simulink model "Battery_Model"  (R2016b)
settings: Solver=ode1  StartTime=0.0  StopTime=1180  FixedStep=0.1  RelTol=1e-3
InitFcn:
  | init_soc=0.6;
values from neighbouring files (symbols this model uses):
  C1_charge = C1_discharge    [Batt_init.m]
  C1_discharge = [54.148429	21.802633	25.586141	30.914925	26.854337	32.525752	40.18035	1.503165	44.76751	43.347833	43.347833 ... (first row only)    [Batt_init.m]
  R0_charge = R0_discharge    [Batt_init.m]
  R0_discharge = [0.0771	0.0168	0.0135	0.0123	0.0117	0.0123	0.0117	0.012	0.0117	0.0114	0.012 ... (first row only)    [Batt_init.m]
  R1_charge = [0.032155	0.008199	0.004763	0.004183	0.00348	0.003242	0.003193	0.003006	0.003091	0.003062	0.003062 ... (first row only)    [Batt_init.m]
  SOC = [0 0.1 0.2 0.3 0.4 0.5 0.6 0.7 0.8 0.9 1]    [Batt_init.m]
  Voc_charge = [2.59 3.22 3.26 3.3 3.3 3.31 3.31 3.32 3.34 3.34 3.47 ... (first row only)    [Batt_init.m]
  Voc_discharge = [2.66	3.19	3.23	3.26	3.28	3.28	3.29	3.3	3.33	3.33	3.4 ... (first row only)    [Batt_init.m]
undefined symbols (not defined in the file or in its folder): cell_capacity, Cp, Hysterisis, Mass_Batt, parallel_cells, series_cells
settings Model: Creator=vguturi  LastModifiedBy=vguturi

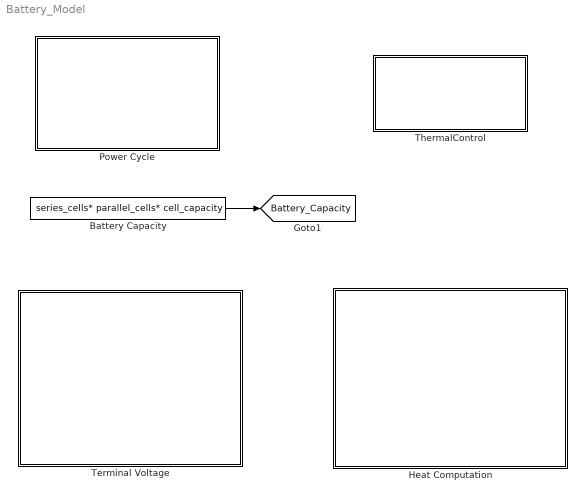
== system Battery_Model ==
  Battery Capacity : Constant  Value=series_cells* parallel_cells* cell_capacity
  Heat Computation : Subsystem  Variant=on  VariantControl=Variant1
  Power Cycle : Subsystem
  Terminal Voltage : Subsystem  Variant=on
  ThermalControl : Subsystem
  tag scope: Battery_Capacity=global
  wires:
  Battery Capacity/1 -> [Battery_Capacity]

== system Battery_Model/Heat Computation ==
  Heat Estimation SimpleR : Subsystem  VariantControl=HeatEst_SimpleR
  Heat Estimation TheveninRC : Subsystem  VariantControl=HeatEst_TheveninRC

== system Battery_Model/Power Cycle ==
  From Workspace : FromWorkspace  VariableName=NEDC
  Scope : Scope
  tag scope: Pd=global
  wires:
  From Workspace/1 -> Scope/1, [Pd]

== system Battery_Model/Terminal Voltage ==
  note: 1) Add Subsystem or Model blocks as valid variant choices.
      | 2) You cannot connect blocks at this level. At simulation, connectivity is automatically
      | determined, based on the active variant and port name matching.
  SimpleResistiveCircuit : Subsystem  VariantControl=SimpleResistive
  TheveninFirstOrder : Subsystem  VariantControl=TheveninRC

== system Battery_Model/ThermalControl ==
  Batt Temp Control : Stateflow chart  TreatAsAtomicUnit=on
  Hysterisis : Constant  Value=Hysterisis
  Scope : Scope  NumInputPorts=2
  tag scope: Cool_Cmd=global
  wires:
  Hysterisis/1 -> Batt Temp Control/1(hysterisis)
  [BattTemp] -> Scope/2, Batt Temp Control/2(Batt_Temp)
  Batt Temp Control/1(Cool_Cmd) -> Scope/1, [Cool_Cmd]

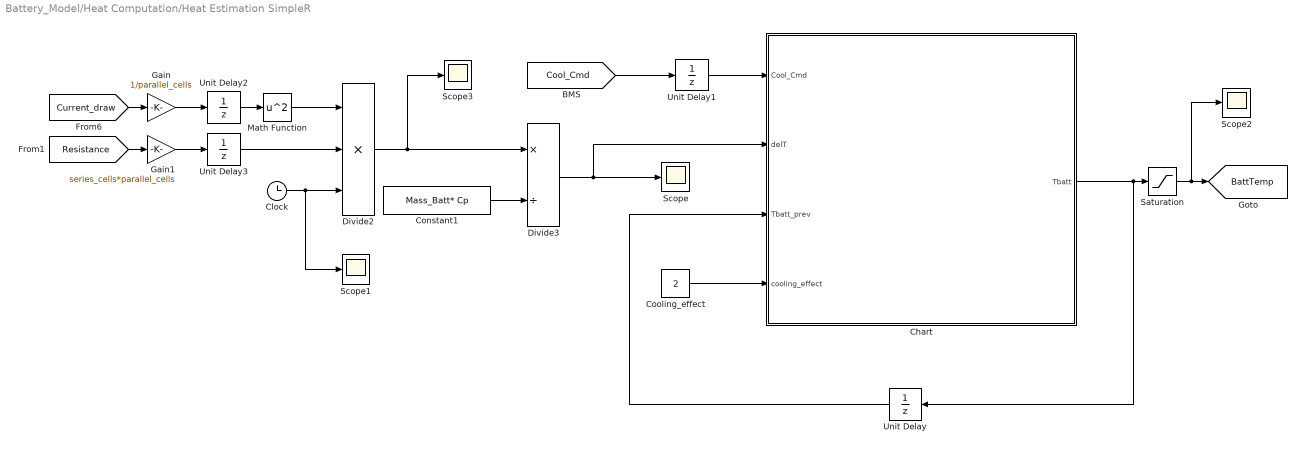
== system Battery_Model/Heat Computation/Heat Estimation SimpleR ==
  Chart : Stateflow chart  TreatAsAtomicUnit=on
  Clock : Clock
  Constant1 : Constant  Value=Mass_Batt* Cp
  Cooling_effect : Constant  Value=2
  Divide2 : Product  Inputs=***
  Divide3 : Product  Inputs=*/
  Gain : Gain  Gain=1/parallel_cells
  Gain1 : Gain  Gain=series_cells*parallel_cells
  Math Function : Math  Operator=square  SaturateOnIntegerOverflow=on
  Saturation : Saturate  UpperLimit=400  LowerLimit=250
  Scope{,1..3} (4 alike) : Scope
  Unit Delay : UnitDelay  InitialCondition=300  SampleTime=-1
  Unit Delay1 : UnitDelay  SampleTime=-1
  Unit Delay2 : UnitDelay  InitialCondition=10  SampleTime=-1
  Unit Delay3 : UnitDelay  InitialCondition=0.012  SampleTime=-1
  tag scope: BattTemp=global
  wires:
  Math Function/1 -> Divide2/1
  Divide2/1 -> Scope3/1, Divide3/1
  [Current_draw] -> Gain/1
  Clock/1 -> Scope1/1, Divide2/3
  Divide3/1 -> Scope/1, Chart/2(delT)
  Constant1/1 -> Divide3/2
  [Resistance] -> Gain1/1
  [Cool_Cmd] -> Unit Delay1/1
  Unit Delay/1 -> Chart/3(Tbatt_prev)
  Chart/1(Tbatt) -> Unit Delay/1, Saturation/1
  Unit Delay1/1 -> Chart/1(Cool_Cmd)
  Cooling_effect/1 -> Chart/4(cooling_effect)
  Unit Delay2/1 -> Math Function/1
  Unit Delay3/1 -> Divide2/2
  Gain/1 -> Unit Delay2/1
  Gain1/1 -> Unit Delay3/1
  Saturation/1 -> Scope2/1, [BattTemp]

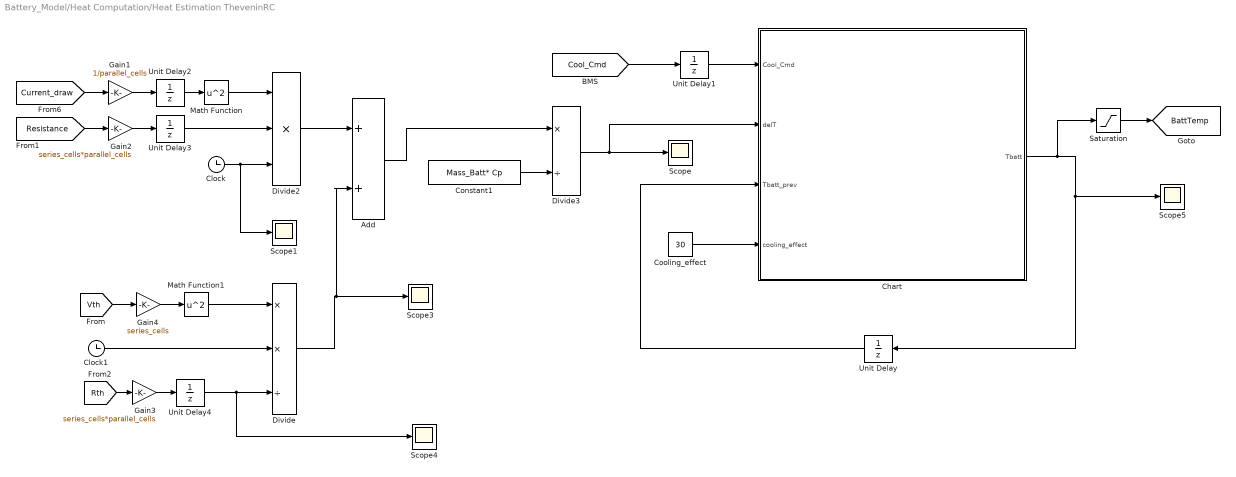
== system Battery_Model/Heat Computation/Heat Estimation TheveninRC ==
  Add : Sum
  Chart : Stateflow chart  TreatAsAtomicUnit=on
  Clock : Clock
  Clock1 : Clock
  Constant1 : Constant  Value=Mass_Batt* Cp
  Cooling_effect : Constant  Value=30
  Divide : Product  Inputs=**/
  Divide2 : Product  Inputs=***
  Divide3 : Product  Inputs=*/
  Gain1 : Gain  Gain=1/parallel_cells
  Gain2 : Gain  Gain=series_cells*parallel_cells
  Gain3 : Gain  Gain=series_cells*parallel_cells
  Gain4 : Gain  Gain=series_cells
  Math Function : Math  Operator=square  SaturateOnIntegerOverflow=on
  Math Function1 : Math  Operator=square  SaturateOnIntegerOverflow=on
  Saturation : Saturate  UpperLimit=400  LowerLimit=250
  Scope{,1,3..5} (5 alike) : Scope
  Unit Delay : UnitDelay  InitialCondition=300  SampleTime=-1
  Unit Delay1 : UnitDelay  SampleTime=-1
  Unit Delay2 : UnitDelay  SampleTime=-1
  Unit Delay3 : UnitDelay  InitialCondition=0.012  SampleTime=-1
  Unit Delay4 : UnitDelay  InitialCondition=0.012  SampleTime=-1
  tag scope: BattTemp=global
  wires:
  Math Function/1 -> Divide2/1
  [Current_draw] -> Gain1/1
  Clock/1 -> Scope1/1, Divide2/3
  Divide3/1 -> Scope/1, Chart/2(delT)
  Constant1/1 -> Divide3/2
  [Resistance] -> Gain2/1
  [Cool_Cmd] -> Unit Delay1/1
  Unit Delay/1 -> Chart/3(Tbatt_prev)
  Chart/1(Tbatt) -> Saturation/1, Scope5/1, Unit Delay/1
  Unit Delay1/1 -> Chart/1(Cool_Cmd)
  Cooling_effect/1 -> Chart/4(cooling_effect)
  Unit Delay2/1 -> Math Function/1
  Unit Delay3/1 -> Divide2/2
  [Vth] -> Gain4/1
  Math Function1/1 -> Divide/1
  [Rth] -> Gain3/1
  Clock1/1 -> Divide/2
  Unit Delay4/1 -> Scope4/1, Divide/3
  Divide2/1 -> Add/1
  Add/1 -> Divide3/1
  Divide/1 -> Add/2, Scope3/1
  Gain2/1 -> Unit Delay3/1
  Gain1/1 -> Unit Delay2/1
  Gain3/1 -> Unit Delay4/1
  Gain4/1 -> Math Function1/1
  Saturation/1 -> [BattTemp]

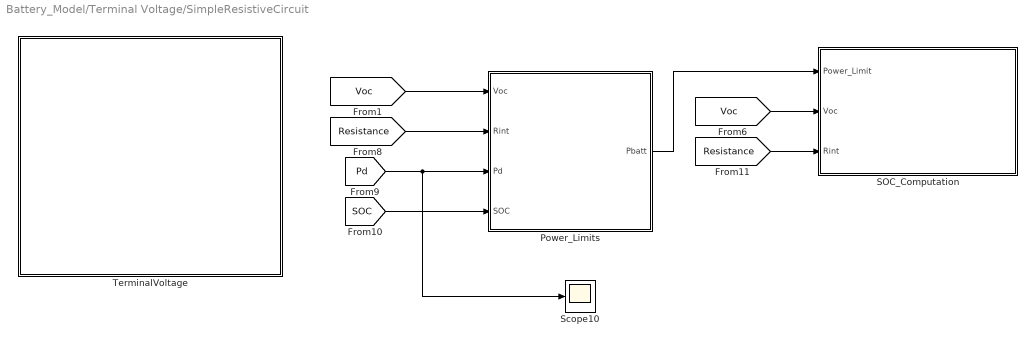
== system Battery_Model/Terminal Voltage/SimpleResistiveCircuit ==
  Power_Limits : Subsystem
  SOC_Computation : Subsystem
  Scope10 : Scope
  TerminalVoltage : Subsystem
  wires:
  [Resistance] -> Power_Limits/2(Rint)
  [Pd] -> Scope10/1, Power_Limits/3(Pd)
  [SOC] -> Power_Limits/4(SOC)
  [Resistance] -> SOC_Computation/3(Rint)
  [Voc] -> Power_Limits/1(Voc)
  [Voc] -> SOC_Computation/2(Voc)
  Power_Limits/1(Pbatt) -> SOC_Computation/1(Power_Limit)

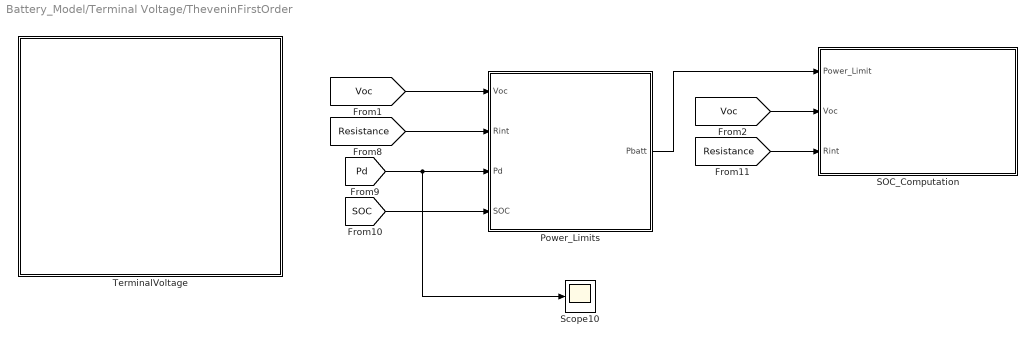
== system Battery_Model/Terminal Voltage/TheveninFirstOrder ==
  Power_Limits : Subsystem
  SOC_Computation : Subsystem
  Scope10 : Scope
  TerminalVoltage : Subsystem
  wires:
  [Resistance] -> Power_Limits/2(Rint)
  [Pd] -> Scope10/1, Power_Limits/3(Pd)
  [SOC] -> Power_Limits/4(SOC)
  [Resistance] -> SOC_Computation/3(Rint)
  [Voc] -> Power_Limits/1(Voc)
  [Voc] -> SOC_Computation/2(Voc)
  Power_Limits/1(Pbatt) -> SOC_Computation/1(Power_Limit)

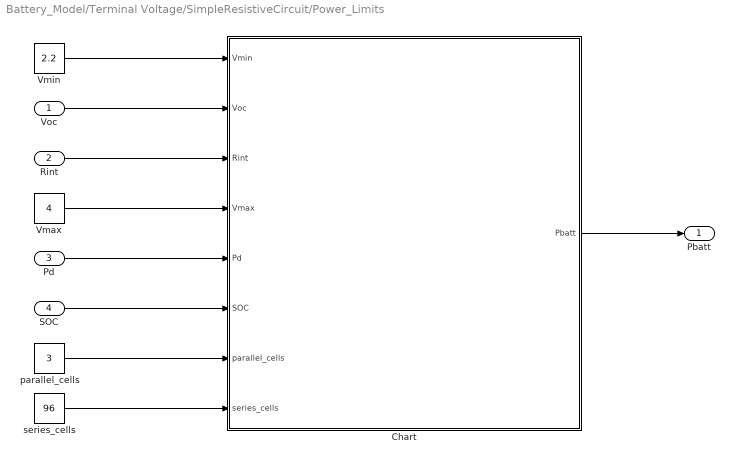
== system Battery_Model/Terminal Voltage/SimpleResistiveCircuit/Power_Limits ==
  Voc : Inport
  Rint : Inport  Port=2
  Pd : Inport  Port=3
  SOC : Inport  Port=4
  Chart : Stateflow chart  TreatAsAtomicUnit=on
  Vmax : Constant  Value=4
  Vmin : Constant  Value=2.2
  parallel_cells : Constant  Value=3
  series_cells : Constant  Value=96
  Pbatt : Outport
  wires:
  Vmin/1 -> Chart/1(Vmin)
  Vmax/1 -> Chart/4(Vmax)
  Voc/1 -> Chart/2(Voc)
  Rint/1 -> Chart/3(Rint)
  Pd/1 -> Chart/5(Pd)
  SOC/1 -> Chart/6(SOC)
  Chart/1(Pbatt) -> Pbatt/1
  series_cells/1 -> Chart/8(series_cells)
  parallel_cells/1 -> Chart/7(parallel_cells)

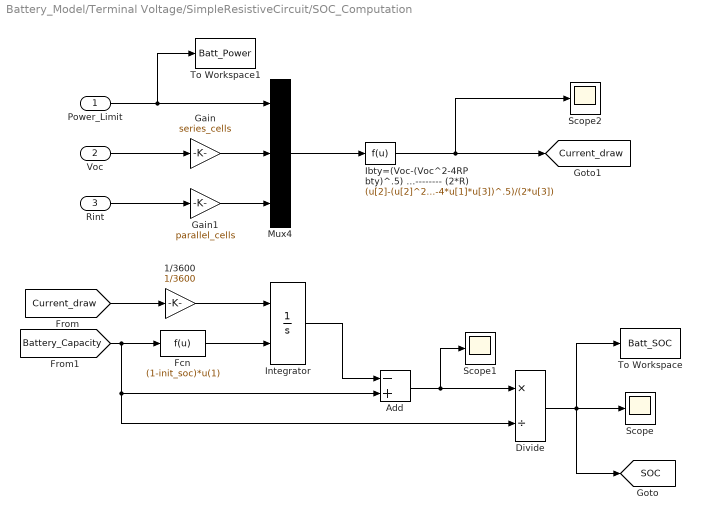
== system Battery_Model/Terminal Voltage/SimpleResistiveCircuit/SOC_Computation ==
  Power_Limit : Inport
  Voc : Inport  Port=2
  Rint : Inport  Port=3
  1/3600 : Gain  Gain=1/3600
  Add : Sum  Inputs=-+
  Divide : Product  Inputs=*/
  Fcn : Fcn  Expr=(1-init_soc)*u(1)
  Gain : Gain  Gain=series_cells
  Gain1 : Gain  Gain=parallel_cells
  Ibty=(Voc-(Voc^2-4RPbty)^.5) ----------------------------- (2*R) : Fcn  Expr=(u[2]-(u[2]^2-4*u[1]*u[3])^.5)/(2*u[3])
  Integrator : Integrator  InitialConditionSource=external
  Mux4 : Mux  Inputs=3
  Scope : Scope
  Scope1 : Scope
  Scope2 : Scope
  To Workspace : ToWorkspace  VariableName=Batt_SOC  SaveFormat=Timeseries  SampleTime=-1
  To Workspace1 : ToWorkspace  VariableName=Batt_Power  SaveFormat=Timeseries  SampleTime=-1
  tag scope: Current_draw=global, SOC=global
  wires:
  1/3600/1 -> Integrator/1
  [Current_draw] -> 1/3600/1
  [Battery_Capacity] -> Fcn/1, Divide/2, Add/2
  Add/1 -> Scope1/1, Divide/1
  Divide/1 -> To Workspace/1, [SOC], Scope/1
  Integrator/1 -> Add/1
  Fcn/1 -> Integrator/2
  Mux4/1 -> Ibty=(Voc-(Voc^2-4RPbty)^.5) ----------------------------- (2*R)/1
  Gain/1 -> Mux4/2
  Gain1/1 -> Mux4/3
  Ibty=(Voc-(Voc^2-4RPbty)^.5) ----------------------------- (2*R)/1 -> Scope2/1, [Current_draw]
  Power_Limit/1 -> To Workspace1/1, Mux4/1
  Voc/1 -> Gain/1
  Rint/1 -> Gain1/1

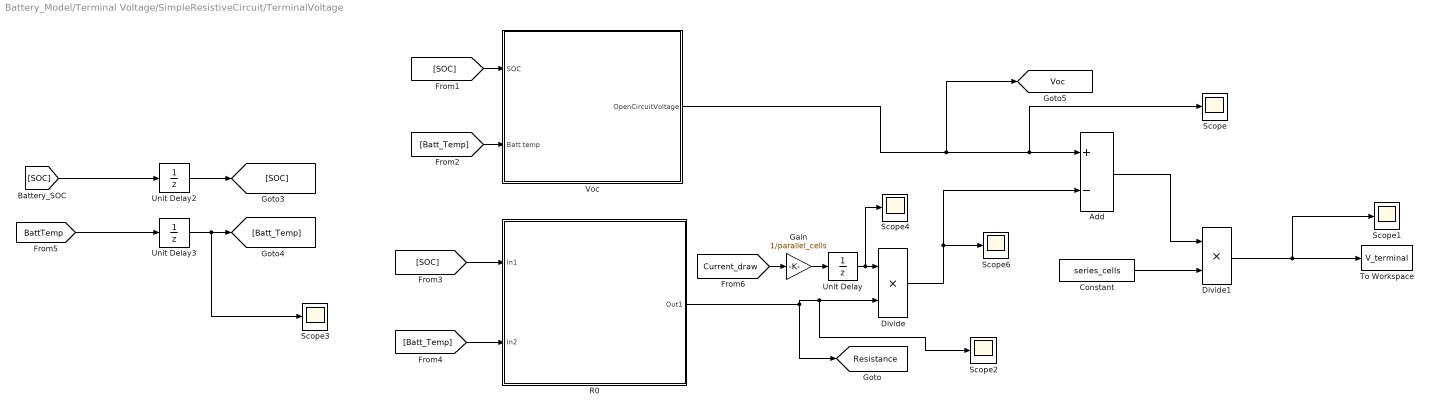
== system Battery_Model/Terminal Voltage/SimpleResistiveCircuit/TerminalVoltage ==
  Add : Sum  Inputs=+-
  Constant : Constant  Value=series_cells
  Divide : Product  Inputs=**
  Divide1 : Product  Inputs=**
  Gain : Gain  Gain=1/parallel_cells
  R0 : Subsystem
  Scope{,1..4,6} (6 alike) : Scope
  To Workspace : ToWorkspace  VariableName=V_terminal  SaveFormat=Timeseries  SampleTime=-1
  Unit Delay : UnitDelay  SampleTime=-1
  Unit Delay2 : UnitDelay  InitialCondition=0.6  SampleTime=-1
  Unit Delay3 : UnitDelay  InitialCondition=300  SampleTime=-1
  Voc : Subsystem
  tag scope: Resistance=global, Voc=global
  wires:
  [SOC] -> Voc/1(SOC)
  [Batt_Temp] -> Voc/2(Batt temp)
  Unit Delay/1 -> Scope4/1, Divide/1
  Add/1 -> Divide1/1
  Divide1/1 -> Scope1/1, To Workspace/1
  Divide/1 -> Scope6/1, Add/2
  Constant/1 -> Divide1/2
  R0/1(Out1) -> Scope2/1, Divide/2, [Resistance]
  [BattTemp] -> Unit Delay3/1
  [SOC] -> Unit Delay2/1
  Unit Delay2/1 -> [SOC]
  Unit Delay3/1 -> Scope3/1, [Batt_Temp]
  [SOC] -> R0/1(In1)
  [Batt_Temp] -> R0/2(In2)
  Voc/1(OpenCircuitVoltage) -> [Voc], Scope/1, Add/1
  [Current_draw] -> Gain/1
  Gain/1 -> Unit Delay/1

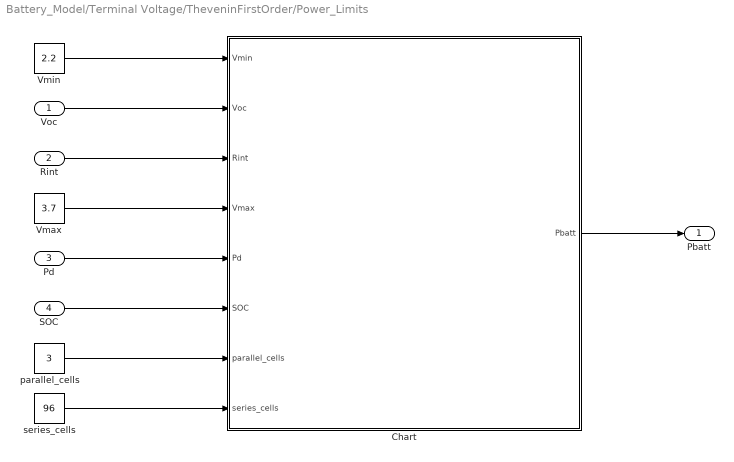
== system Battery_Model/Terminal Voltage/TheveninFirstOrder/Power_Limits ==
  Voc : Inport
  Rint : Inport  Port=2
  Pd : Inport  Port=3
  SOC : Inport  Port=4
  Chart : Stateflow chart  TreatAsAtomicUnit=on
  Vmax : Constant  Value=3.7
  Vmin : Constant  Value=2.2
  parallel_cells : Constant  Value=3
  series_cells : Constant  Value=96
  Pbatt : Outport
  wires:
  Vmin/1 -> Chart/1(Vmin)
  Vmax/1 -> Chart/4(Vmax)
  Voc/1 -> Chart/2(Voc)
  Rint/1 -> Chart/3(Rint)
  Pd/1 -> Chart/5(Pd)
  SOC/1 -> Chart/6(SOC)
  Chart/1(Pbatt) -> Pbatt/1
  series_cells/1 -> Chart/8(series_cells)
  parallel_cells/1 -> Chart/7(parallel_cells)

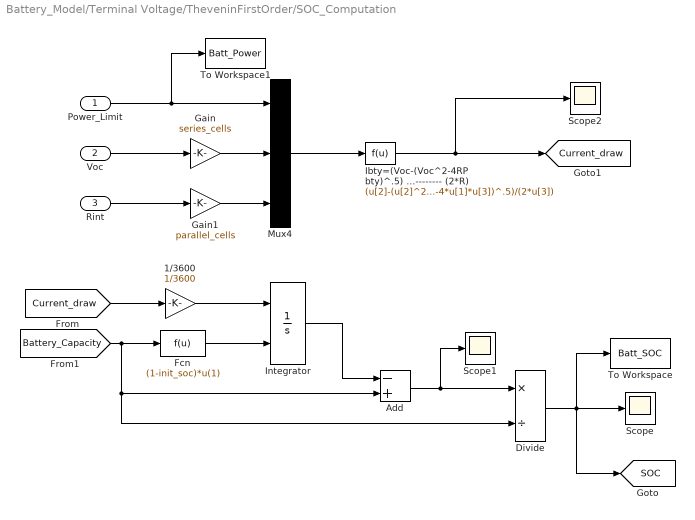
== system Battery_Model/Terminal Voltage/TheveninFirstOrder/SOC_Computation ==
  Power_Limit : Inport
  Voc : Inport  Port=2
  Rint : Inport  Port=3
  1/3600 : Gain  Gain=1/3600
  Add : Sum  Inputs=-+
  Divide : Product  Inputs=*/
  Fcn : Fcn  Expr=(1-init_soc)*u(1)
  Gain : Gain  Gain=series_cells
  Gain1 : Gain  Gain=parallel_cells
  Ibty=(Voc-(Voc^2-4RPbty)^.5) ----------------------------- (2*R) : Fcn  Expr=(u[2]-(u[2]^2-4*u[1]*u[3])^.5)/(2*u[3])
  Integrator : Integrator  InitialConditionSource=external
  Mux4 : Mux  Inputs=3
  Scope : Scope
  Scope1 : Scope
  Scope2 : Scope
  To Workspace : ToWorkspace  VariableName=Batt_SOC  SaveFormat=Timeseries  SampleTime=-1
  To Workspace1 : ToWorkspace  VariableName=Batt_Power  SaveFormat=Timeseries  SampleTime=-1
  tag scope: Current_draw=global, SOC=global
  wires:
  1/3600/1 -> Integrator/1
  [Current_draw] -> 1/3600/1
  [Battery_Capacity] -> Fcn/1, Divide/2, Add/2
  Add/1 -> Scope1/1, Divide/1
  Divide/1 -> To Workspace/1, [SOC], Scope/1
  Integrator/1 -> Add/1
  Fcn/1 -> Integrator/2
  Mux4/1 -> Ibty=(Voc-(Voc^2-4RPbty)^.5) ----------------------------- (2*R)/1
  Gain/1 -> Mux4/2
  Gain1/1 -> Mux4/3
  Ibty=(Voc-(Voc^2-4RPbty)^.5) ----------------------------- (2*R)/1 -> Scope2/1, [Current_draw]
  Power_Limit/1 -> To Workspace1/1, Mux4/1
  Voc/1 -> Gain/1
  Rint/1 -> Gain1/1

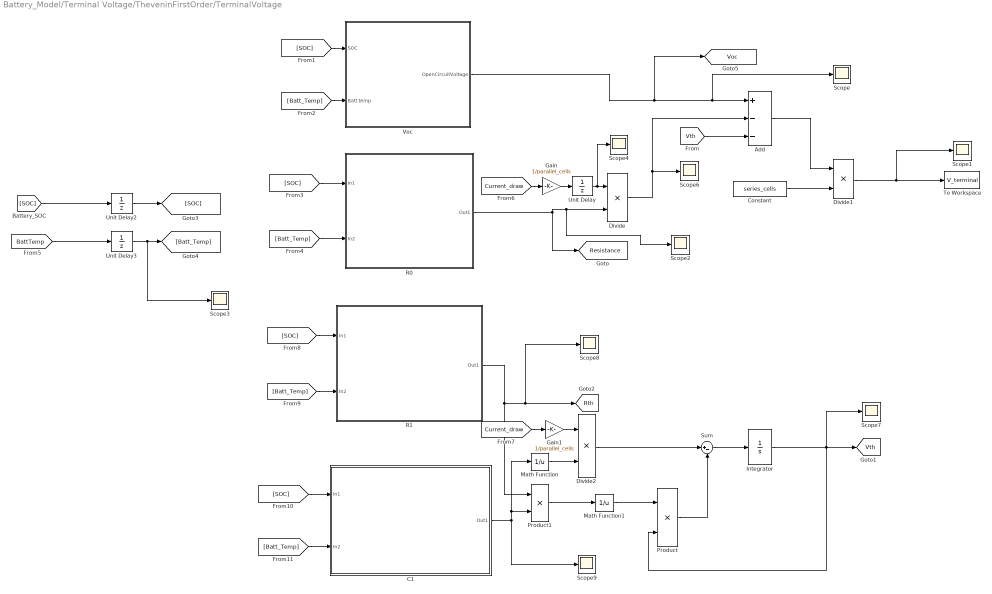
== system Battery_Model/Terminal Voltage/TheveninFirstOrder/TerminalVoltage ==
  Add : Sum  Inputs=+--
  C1 : Subsystem
  Constant : Constant  Value=series_cells
  Divide : Product  Inputs=**
  Divide1 : Product  Inputs=**
  Divide2 : Product  Inputs=**
  Gain : Gain  Gain=1/parallel_cells
  Gain1 : Gain  Gain=1/parallel_cells
  Integrator : Integrator
  Math Function : Math  Operator=reciprocal  SaturateOnIntegerOverflow=on
  Math Function1 : Math  Operator=reciprocal  SaturateOnIntegerOverflow=on
  Product : Product
  Product1 : Product
  R0 : Subsystem
  R1 : Subsystem
  Scope{,1..4,6..9} (9 alike) : Scope
  Sum : Sum  Inputs=|+-
  To Workspace : ToWorkspace  VariableName=V_terminal  SaveFormat=Timeseries  SampleTime=-1
  Unit Delay : UnitDelay  SampleTime=-1
  Unit Delay2 : UnitDelay  InitialCondition=0.6  SampleTime=-1
  Unit Delay3 : UnitDelay  InitialCondition=300  SampleTime=-1
  Voc : Subsystem
  tag scope: Resistance=global, Rth=global, Voc=global, Vth=global
  wires:
  [SOC] -> R1/1(In1)
  [SOC] -> Voc/1(SOC)
  [Batt_Temp] -> Voc/2(Batt temp)
  [Batt_Temp] -> R1/2(In2)
  Unit Delay/1 -> Scope4/1, Divide/1
  Add/1 -> Divide1/1
  Divide1/1 -> Scope1/1, To Workspace/1
  Divide/1 -> Scope6/1, Add/2
  Constant/1 -> Divide1/2
  Integrator/1 -> Scope7/1, [Vth], Product/2
  [Current_draw] -> Gain1/1
  Math Function/1 -> Divide2/2
  [Vth] -> Add/3
  Product1/1 -> Math Function1/1
  Product/1 -> Sum/2
  Math Function1/1 -> Product/1
  Sum/1 -> Integrator/1
  Divide2/1 -> Sum/1
  R0/1(Out1) -> Scope2/1, Divide/2, [Resistance]
  R1/1(Out1) -> Product1/1, Scope8/1, [Rth]
  C1/1(Out1) -> Scope9/1, Math Function/1, Product1/2
  [BattTemp] -> Unit Delay3/1
  [SOC] -> Unit Delay2/1
  Unit Delay2/1 -> [SOC]
  Unit Delay3/1 -> Scope3/1, [Batt_Temp]
  [SOC] -> R0/1(In1)
  [Batt_Temp] -> R0/2(In2)
  [SOC] -> C1/1(In1)
  [Batt_Temp] -> C1/2(In2)
  Voc/1(OpenCircuitVoltage) -> [Voc], Scope/1, Add/1
  [Current_draw] -> Gain/1
  Gain/1 -> Unit Delay/1
  Gain1/1 -> Divide2/1

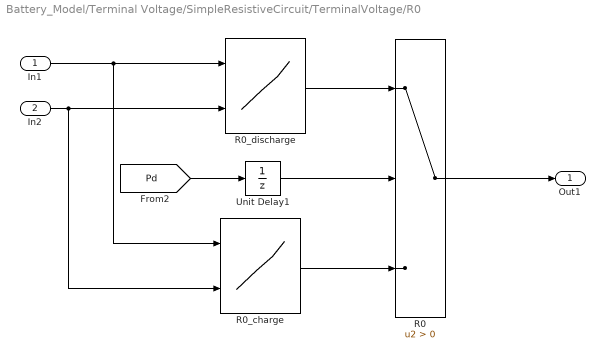
== system Battery_Model/Terminal Voltage/SimpleResistiveCircuit/TerminalVoltage/R0 ==
  In1 : Inport
  In2 : Inport  Port=2
  R0 : Switch  Criteria=u2 > Threshold
  R0_charge : Lookup_n-D  BreakpointsForDimension1=[293 303 313]  BreakpointsForDimension2=SOC  Table=R0_charge  ExtrapMethod=Clip  UseLastTableValue=on  InternalRulePriority=Speed  RndMeth=Simplest  InputSameDT=on
  R0_discharge : Lookup_n-D  BreakpointsForDimension1=[293 303 313]  BreakpointsForDimension2=SOC  Table=R0_discharge  ExtrapMethod=Clip  UseLastTableValue=on  InternalRulePriority=Speed  RndMeth=Simplest  InputSameDT=on
  Unit Delay1 : UnitDelay  SampleTime=-1
  Out1 : Outport
  wires:
  [Pd] -> Unit Delay1/1
  Unit Delay1/1 -> R0/2
  R0_discharge/1 -> R0/1
  R0_charge/1 -> R0/3
  R0/1 -> Out1/1
  In1/1 -> R0_charge/1, R0_discharge/1
  In2/1 -> R0_charge/2, R0_discharge/2

== system Battery_Model/Terminal Voltage/SimpleResistiveCircuit/TerminalVoltage/Voc ==
  SOC : Inport
  Batt temp : Inport  Port=2
  Voc : Switch  Criteria=u2 > Threshold
  Voc_charge : Lookup_n-D  BreakpointsForDimension1=[293 303 313]  BreakpointsForDimension2=SOC  Table=Voc_charge  ExtrapMethod=Clip  UseLastTableValue=on  InternalRulePriority=Speed  RndMeth=Simplest  InputSameDT=on
  Voc_discharge : Lookup_n-D  BreakpointsForDimension1=[293 303 313]  BreakpointsForDimension2=SOC  Table=Voc_discharge  ExtrapMethod=Clip  UseLastTableValue=on  InternalRulePriority=Speed  RndMeth=Simplest  InputSameDT=on
  OpenCircuitVoltage : Outport
  wires:
  Batt temp/1 -> Voc_charge/2, Voc_discharge/2
  SOC/1 -> Voc_discharge/1, Voc_charge/1
  Voc_charge/1 -> Voc/3
  Voc/1 -> OpenCircuitVoltage/1
  [Pd] -> Voc/2
  Voc_discharge/1 -> Voc/1

== system Battery_Model/Terminal Voltage/TheveninFirstOrder/TerminalVoltage/C1 ==
  In1 : Inport
  In2 : Inport  Port=2
  C1 : Switch  Criteria=u2 > Threshold
  C1_charge : Lookup_n-D  BreakpointsForDimension1=[293 303 313]  BreakpointsForDimension2=SOC  Table=C1_charge  ExtrapMethod=Clip  UseLastTableValue=on  InternalRulePriority=Speed  RndMeth=Simplest  InputSameDT=on
  C1_discharge : Lookup_n-D  BreakpointsForDimension1=[293 303 313]  BreakpointsForDimension2=SOC  Table=C1_discharge  ExtrapMethod=Clip  UseLastTableValue=on  InternalRulePriority=Speed  RndMeth=Simplest  InputSameDT=on
  Unit Delay5 : UnitDelay  SampleTime=-1
  Out1 : Outport
  wires:
  [Pd] -> Unit Delay5/1
  Unit Delay5/1 -> C1/2
  C1_discharge/1 -> C1/1
  C1_charge/1 -> C1/3
  C1/1 -> Out1/1
  In1/1 -> C1_charge/1, C1_discharge/1
  In2/1 -> C1_charge/2, C1_discharge/2

== system Battery_Model/Terminal Voltage/TheveninFirstOrder/TerminalVoltage/R0 ==
  In1 : Inport
  In2 : Inport  Port=2
  R0 : Switch  Criteria=u2 > Threshold
  R0_charge : Lookup_n-D  BreakpointsForDimension1=[293 303 313]  BreakpointsForDimension2=SOC  Table=R0_charge  ExtrapMethod=Clip  UseLastTableValue=on  InternalRulePriority=Speed  RndMeth=Simplest  InputSameDT=on
  R0_discharge : Lookup_n-D  BreakpointsForDimension1=[293 303 313]  BreakpointsForDimension2=SOC  Table=R0_discharge  ExtrapMethod=Clip  UseLastTableValue=on  InternalRulePriority=Speed  RndMeth=Simplest  InputSameDT=on
  Unit Delay1 : UnitDelay  SampleTime=-1
  Out1 : Outport
  wires:
  [Pd] -> Unit Delay1/1
  Unit Delay1/1 -> R0/2
  R0_discharge/1 -> R0/1
  R0_charge/1 -> R0/3
  R0/1 -> Out1/1
  In1/1 -> R0_charge/1, R0_discharge/1
  In2/1 -> R0_charge/2, R0_discharge/2

== system Battery_Model/Terminal Voltage/TheveninFirstOrder/TerminalVoltage/R1 ==
  In1 : Inport
  In2 : Inport  Port=2
  R1 : Switch  Criteria=u2 > Threshold
  R1_charge : Lookup_n-D  BreakpointsForDimension1=[293 303 313]  BreakpointsForDimension2=SOC  Table=R1_charge  ExtrapMethod=Clip  UseLastTableValue=on  InternalRulePriority=Speed  RndMeth=Simplest  InputSameDT=on
  R1_discharge : Lookup_n-D  BreakpointsForDimension1=[293 303 313]  BreakpointsForDimension2=SOC  Table=R0_discharge  ExtrapMethod=Clip  UseLastTableValue=on  InternalRulePriority=Speed  RndMeth=Simplest  InputSameDT=on
  Unit Delay4 : UnitDelay  SampleTime=-1
  Out1 : Outport
  wires:
  Unit Delay4/1 -> R1/2
  [Pd] -> Unit Delay4/1
  R1_charge/1 -> R1/3
  R1_discharge/1 -> R1/1
  R1/1 -> Out1/1
  In1/1 -> R1_charge/1, R1_discharge/1
  In2/1 -> R1_charge/2, R1_discharge/2

== system Battery_Model/Terminal Voltage/TheveninFirstOrder/TerminalVoltage/Voc ==
  SOC : Inport
  Batt temp : Inport  Port=2
  Voc : Switch  Criteria=u2 > Threshold
  Voc_charge : Lookup_n-D  BreakpointsForDimension1=[293 303 313]  BreakpointsForDimension2=SOC  Table=Voc_charge  ExtrapMethod=Clip  UseLastTableValue=on  InternalRulePriority=Speed  RndMeth=Simplest  InputSameDT=on
  Voc_discharge : Lookup_n-D  BreakpointsForDimension1=[293 303 313]  BreakpointsForDimension2=SOC  Table=Voc_discharge  ExtrapMethod=Clip  UseLastTableValue=on  InternalRulePriority=Speed  RndMeth=Simplest  InputSameDT=on
  OpenCircuitVoltage : Outport
  wires:
  Batt temp/1 -> Voc_charge/2, Voc_discharge/2
  SOC/1 -> Voc_discharge/1, Voc_charge/1
  Voc_charge/1 -> Voc/3
  Voc/1 -> OpenCircuitVoltage/1
  [Pd] -> Voc/2
  Voc_discharge/1 -> Voc/1

== stateflow chart Battery_Model/ThermalControl/Batt Temp Control ==
  state OFF
    during:
    Cool_Cmd = 0 ;
  state ON
    during:
    Cool_Cmd = 1;
  (default) -> OFF
  OFF -> ON : [Batt_Temp > 325 + hysterisis ]
  ON -> OFF : [Batt_Temp < 325 - hysterisis]
  data: hysterisis input; Batt_Temp input; Cool_Cmd output

== stateflow chart Battery_Model/Heat Computation/Heat Estimation TheveninRC/Chart ==
  state OFF
    during:
    Tbatt = Tbatt_prev + delT;
  state ON
    during :
    Tbatt = Tbatt_prev - cooling_effect;
  (default) -> OFF : {Tbatt =300;}
  OFF -> ON : [Cool_Cmd == 1]
  ON -> OFF : [Cool_Cmd == 0]
  data: Tbatt output; Cool_Cmd input; delT input; Tbatt_prev input; cooling_effect input

== stateflow chart Battery_Model/Heat Computation/Heat Estimation SimpleR/Chart ==
  state OFF
    during:
    Tbatt = Tbatt_prev + delT;
  state ON
    during :
    Tbatt = Tbatt_prev - cooling_effect;
  (default) -> OFF : {Tbatt =300;}
  OFF -> ON : [Cool_Cmd == 1]
  ON -> OFF : [Cool_Cmd == 0]
  data: Tbatt output; Cool_Cmd input; delT input; Tbatt_prev input; cooling_effect input

== stateflow chart Battery_Model/Terminal Voltage/TheveninFirstOrder/Power_Limits/Chart ==
  state No_Discharge
    during:
    Pbatt = 0;
  state Discharge
    during:
    Pcell= Vmin * (Voc - Vmin)/Rint;
    Pbatt = min(Pd,Pcell*series_cells*parallel_cells);
  state Charge
    during:
    Pcell = Vmax*(Vmax - Voc)/Rint;
    Pbatt = min(abs(Pd),Pcell * series_cells*parallel_cells);
  state No_Charge
    during:
    Pbatt =0;
  (default) -> Discharge
  Discharge -> No_Discharge [order 2] : [SOC <= 0 ]
  Discharge -> Charge [order 1] : [Pd<0]
  Charge -> Discharge [order 1] : [Pd>=0]
  Charge -> No_Charge [order 2] : [SOC> 0.99]
  data: Vmin input; Voc input; Rint input; Vmax input; Pd input; Pbatt output; SOC input; Pcell local; parallel_cells input; series_cells input

== stateflow chart Battery_Model/Terminal Voltage/SimpleResistiveCircuit/Power_Limits/Chart ==
  state No_Discharge
    during:
    Pbatt = 0;
  state Discharge
    during:
    Pcell= Vmin * (Voc - Vmin)/Rint;
    Pbatt = min(Pd,Pcell*series_cells*parallel_cells);
  state Charge
    during:
    Pcell = Vmax*(Vmax - Voc)/Rint;
    Pbatt = max(Pd,Pcell * series_cells*parallel_cells);
  state No_Charge
    during:
    Pbatt =0;
  (default) -> Discharge
  Discharge -> No_Discharge [order 2] : [SOC <= 0 ]
  Discharge -> Charge [order 1] : [Pd<0]
  Charge -> Discharge [order 1] : [Pd>=0]
  Charge -> No_Charge [order 2] : [SOC> 0.99]
  data: Vmin input; Voc input; Rint input; Vmax input; Pd input; Pbatt output; SOC input; Pcell local; parallel_cells input; series_cells input
